simulink model "project_simulation"  (R2018a)
settings: Solver=VariableStepAuto  StartTime=0.0  StopTime=10.0  RelTol=1e-3
values from neighbouring files (symbols this model uses):
  a = [0 1 ; 0 -6.523]    [Project_state_space.m]
  b = [0;1]    [Project_state_space.m]
  c = [0.09667 0]    [Project_state_space.m]
  k = place(sysssD.a,sysssD.b,[0.9 0.7])    [Discret_LEGO_script.m]    (also in Project_state_space.m = place(a, b, P'); RLS_Glemselsfaktor.m = Q*Phi'; RLS_Kalman.m = Q*Phi'; RLS_Online.m = p*Phi')
  L = [l1; l2]    [Project_state_space.m]
settings Model: Creator=Lenovo  LastModifiedBy=Lenovo

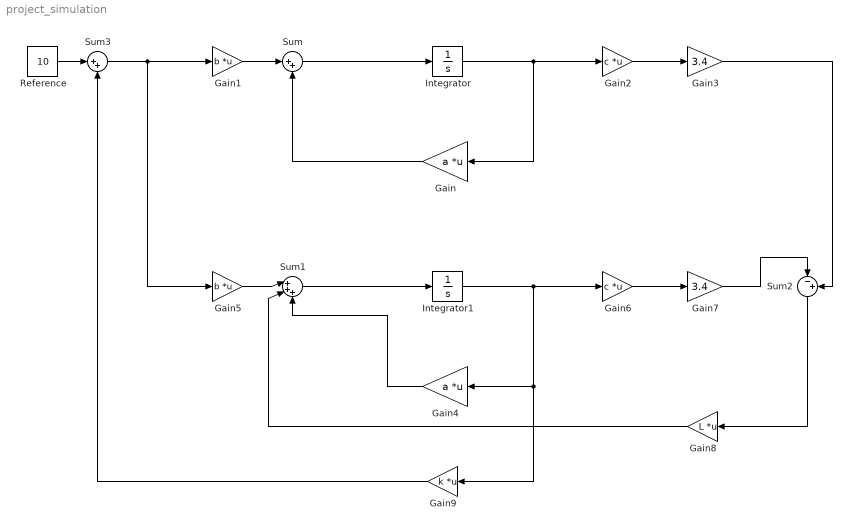
== system project_simulation ==
  Gain : Gain  Gain=a  Multiplication=Matrix(K*u)
  Gain1 : Gain  Gain=b  Multiplication=Matrix(K*u)
  Gain2 : Gain  Gain=c  Multiplication=Matrix(K*u)
  Gain3 : Gain  Gain=3.4
  Gain4 : Gain  Gain=a  Multiplication=Matrix(K*u)
  Gain5 : Gain  Gain=b  Multiplication=Matrix(K*u)
  Gain6 : Gain  Gain=c  Multiplication=Matrix(K*u)
  Gain7 : Gain  Gain=3.4
  Gain8 : Gain  Gain=L  Multiplication=Matrix(K*u)
  Gain9 : Gain  Gain=k  Multiplication=Matrix(K*u)
  Integrator : Integrator
  Integrator1 : Integrator
  Reference : Constant  Value=10
  Sum : Sum  Inputs=|++
  Sum1 : Sum  Inputs=|+++
  Sum2 : Sum  Inputs=|-+
  Sum3 : Sum  Inputs=|++
  wires:
  Sum/1 -> Integrator/1
  Integrator/1 -> Gain/1, Gain2/1
  Gain/1 -> Sum/2
  Gain1/1 -> Sum/1
  Gain2/1 -> Gain3/1
  Gain3/1 -> Sum2/2
  Gain4/1 -> Sum1/3
  Integrator1/1 -> Gain9/1, Gain4/1, Gain6/1
  Sum1/1 -> Integrator1/1
  Gain5/1 -> Sum1/1
  Gain7/1 -> Sum2/1
  Gain6/1 -> Gain7/1
  Sum2/1 -> Gain8/1
  Gain8/1 -> Sum1/2
  Gain9/1 -> Sum3/2
  Sum3/1 -> Gain5/1, Gain1/1
  Reference/1 -> Sum3/1
